simulink model "ADC_Capture_4x4_IQ_DDR4"  (R2019b)
settings: Solver=FixedStepDiscrete  StartTime=0.0  StopTime=inf  RelTol=1e-3
InitFcn:
  | init_ADC_Capture_4x4_IQ_DDR4
values from neighbouring files (symbols this model uses):
  Fs = ConverterSamplingRate/DDC_DUC_factor    (= 512000000)    [init_ADC_Capture_4x4_IQ_DDR4.m]
  N = 14    [init_ADC_Capture_4x4_IQ_DDR4.m]
  sim_CaptureLength = CaptureLength    (= 4096)    [init_ADC_Capture_4x4_IQ_DDR4.m]
  sim_RdFrameSize = 64    [init_ADC_Capture_4x4_IQ_DDR4.m]
  sim_RdNumFrames = ceil(sim_CaptureLength/sim_RdFrameSize)    [init_ADC_Capture_4x4_IQ_DDR4.m]
undefined symbols (not defined in the file or in its folder): config, DDR, Fo
libraries: hdlsllib x35, simulink x20, ddr4_behavioral_mdl x1, AXIDMALib x1, dsphdlsigops x1
(part 2 of 3)

== system ADC_Capture_4x4_IQ_DDR4/HDL_IP/DefaultRegister2 ==
  note: Give it default non-zero value at start-up time
  In1 : Inport
  Compare To Zero : simulink/Logic and Bit Operations/Compare To Zero  relop===  OutDataTypeStr=boolean
  Delay1 : Delay  DelayLength=1
  Switch2 : Switch  Criteria=u2 > Threshold
  range swath cycles : Constant  Value=config.register.range_swath_cycles  OutDataTypeStr=uint32  SampleTime=-1
  Out2 : Outport  VectorParamsAs1DForOutWhenUnconnected=off
  wires:
  In1/1 -> Delay1/1
  range swath cycles/1 -> Switch2/1
  Delay1/1 -> Switch2/3, Compare To Zero/1
  Switch2/1 -> Out2/1
  Compare To Zero/1 -> Switch2/2

== system ADC_Capture_4x4_IQ_DDR4/HDL_IP/DefaultRegister3 ==
  note: Give it default non-zero value at start-up time
  In1 : Inport
  Compare To Zero : simulink/Logic and Bit Operations/Compare To Zero  relop===  OutDataTypeStr=boolean
  Delay1 : Delay  DelayLength=1
  Switch2 : Switch  Criteria=u2 > Threshold
  tx end to rx start cycles : Constant  Value=config.register.tx_end_to_rx_start_delay_cycles  OutDataTypeStr=uint32  SampleTime=-1
  Out2 : Outport  VectorParamsAs1DForOutWhenUnconnected=off
  wires:
  In1/1 -> Delay1/1
  tx end to rx start cycles/1 -> Switch2/1
  Delay1/1 -> Switch2/3, Compare To Zero/1
  Switch2/1 -> Out2/1
  Compare To Zero/1 -> Switch2/2

== system ADC_Capture_4x4_IQ_DDR4/HDL_IP/DefaultRegister4 ==
  note: Give it default non-zero value at start-up time
  In1 : Inport
  Compare To Zero : simulink/Logic and Bit Operations/Compare To Zero  relop===  OutDataTypeStr=boolean
  Constant5 : Constant  Value=config.register.pri_cycles  OutDataTypeStr=uint32  SampleTime=-1
  Delay1 : Delay  DelayLength=1
  Switch2 : Switch  Criteria=u2 > Threshold
  Out2 : Outport  VectorParamsAs1DForOutWhenUnconnected=off
  wires:
  In1/1 -> Delay1/1
  Constant5/1 -> Switch2/1
  Delay1/1 -> Switch2/3, Compare To Zero/1
  Switch2/1 -> Out2/1
  Compare To Zero/1 -> Switch2/2

== system ADC_Capture_4x4_IQ_DDR4/HDL_IP/DefaultRegister5 ==
  note: Give it default non-zero value at start-up time
  In1 : Inport
  Compare To Zero : simulink/Logic and Bit Operations/Compare To Zero  relop===  OutDataTypeStr=boolean
  Constant5 : Constant  Value=config.register.pulse_width_cycles  OutDataTypeStr=uint32  SampleTime=-1
  Delay1 : Delay  DelayLength=1
  Switch2 : Switch  Criteria=u2 > Threshold
  Out2 : Outport  VectorParamsAs1DForOutWhenUnconnected=off
  wires:
  In1/1 -> Delay1/1
  Constant5/1 -> Switch2/1
  Delay1/1 -> Switch2/3, Compare To Zero/1
  Switch2/1 -> Out2/1
  Compare To Zero/1 -> Switch2/2

== system ADC_Capture_4x4_IQ_DDR4/HDL_IP/DefaultRegister6 ==
  note: Give it default non-zero value at start-up time
  In1 : Inport
  Compare To Zero : simulink/Logic and Bit Operations/Compare To Zero  relop===  OutDataTypeStr=boolean
  Constant5 : Constant  Value=config.radar.pulses_per_cpi  OutDataTypeStr=uint32  SampleTime=-1
  Delay1 : Delay  DelayLength=1
  Switch2 : Switch  Criteria=u2 > Threshold
  Out2 : Outport  VectorParamsAs1DForOutWhenUnconnected=off
  wires:
  In1/1 -> Delay1/1
  Constant5/1 -> Switch2/1
  Delay1/1 -> Switch2/3, Compare To Zero/1
  Switch2/1 -> Out2/1
  Compare To Zero/1 -> Switch2/2

== system ADC_Capture_4x4_IQ_DDR4/HDL_IP/DefaultRegister8 ==
  note: Give it default non-zero value at start-up time
  In1 : Inport
  Compare To Zero : simulink/Logic and Bit Operations/Compare To Zero  relop===  OutDataTypeStr=boolean
  Data Type Conversion : DataTypeConversion  OutDataTypeStr=int32
  Delay1 : Delay  DelayLength=1
  Switch2 : Switch  Criteria=u2 > Threshold  OutDataTypeStr=int32
  start inc steps : Constant  Value=config.register.start_inc_steps  OutDataTypeStr=int32
  Out2 : Outport  VectorParamsAs1DForOutWhenUnconnected=off
  wires:
  Compare To Zero/1 -> Switch2/2
  Switch2/1 -> Out2/1
  Delay1/1 -> Compare To Zero/1, Switch2/3
  Data Type Conversion/1 -> Switch2/1
  In1/1 -> Delay1/1
  start inc steps/1 -> Data Type Conversion/1

== system ADC_Capture_4x4_IQ_DDR4/HDL_IP/DefaultRegister9 ==
  note: Give it default non-zero value at start-up time
  In1 : Inport
  Compare To Zero : simulink/Logic and Bit Operations/Compare To Zero  relop===  OutDataTypeStr=boolean
  Data Type Conversion : DataTypeConversion  OutDataTypeStr=int32
  Delay1 : Delay  DelayLength=1
  Switch2 : Switch  Criteria=u2 > Threshold  OutDataTypeStr=int32
  end_inc_steps : Constant  Value=config.register.end_inc_steps  OutDataTypeStr=int32
  Out2 : Outport  VectorParamsAs1DForOutWhenUnconnected=off
  wires:
  Compare To Zero/1 -> Switch2/2
  Switch2/1 -> Out2/1
  Delay1/1 -> Compare To Zero/1, Switch2/3
  Data Type Conversion/1 -> Switch2/1
  In1/1 -> Delay1/1
  end_inc_steps/1 -> Data Type Conversion/1

== system ADC_Capture_4x4_IQ_DDR4/HDL_IP/GateRxData ==
  active : Inport
  in : Inport  Port=2
  Bus Creator : BusCreator  Inputs=3
  Bus Selector4 : BusSelector  OutputSignals=I,Q,Valid
  Delay : Delay  DelayLength=1
  Delay1 : Delay  DelayLength=1
  Delay2 : Delay  DelayLength=1
  Logical Operator : Logic  AllPortsSameDT=off  OutDataTypeStr=boolean
  Signal Conversion13 : SignalConversion  OverrideOpt=off
  Signal Conversion14 : SignalConversion  OverrideOpt=off
  Signal Conversion15 : SignalConversion  OverrideOpt=off
  out : Outport
  wires:
  in/1 -> Delay1/1
  Bus Selector4/3 -> Logical Operator/1  "<Valid>"
  active/1 -> Delay2/1
  Signal Conversion14/1 -> Bus Creator/2  "Q"
  Signal Conversion15/1 -> Bus Creator/3  "Valid"
  Bus Creator/1 -> Delay/1
  Signal Conversion13/1 -> Bus Creator/1  "I"
  Bus Selector4/1 -> Signal Conversion13/1  "<I>"
  Bus Selector4/2 -> Signal Conversion14/1  "<Q>"
  Logical Operator/1 -> Signal Conversion15/1
  Delay/1 -> out/1
  Delay1/1 -> Bus Selector4/1
  Delay2/1 -> Logical Operator/2

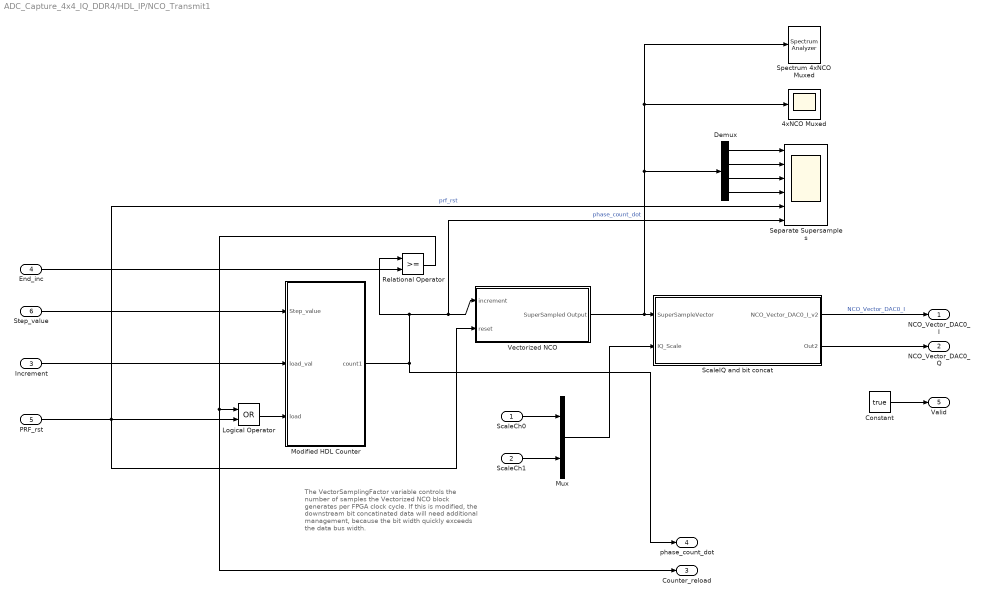
== system ADC_Capture_4x4_IQ_DDR4/HDL_IP/NCO_Transmit1 ==
  note: The VectorSamplingFactor variable controls the
      | number of samples the Vectorized NCO block
      | generates per FPGA clock cycle.
      | If this is modified, the downstream bit concatinated
      | data will need additional management, because
      | the bit width quickly exceeds the data bus width.
  ScaleCh0 : Inport
  ScaleCh1 : Inport  Port=2
  Increment : Inport  Port=3
  End_inc : Inport  Port=4
  PRF_rst : Inport  Port=5
  Step_value : Inport  Port=6
  4xNCO Muxed : Scope
  Constant : Constant  Value=true  SampleTime=-1
  Demux : Demux
  Logical Operator : Logic  Operator=OR  AllPortsSameDT=off  OutDataTypeStr=boolean
  Modified HDL Counter : Subsystem  mask{N=config.synthesis.N_accumulator}
      mask prompts: N "Counter Bit Depth"
      mask init:
      | issigned = 1; % 0 - unsigned, 1 - signed
      | CountInit = 0;
      | CountFracLen = 0;
      | CountWordLen = N;
      | freerun=1;
      | CountFrom = 0;
      | CountDir = 0; % 0-up, 1-down
      | % MaxValue for N bit signed integer
      | MaxValue = 2^(N-1)-1;
  Mux : Mux  Inputs=2
  Relational Operator : RelationalOperator  OutDataTypeStr=boolean  RndMeth=Nearest
  ScaleIQ and bit concat : Subsystem
  Separate Supersamples : Scope  NumInputPorts=6
  Spectrum 4xNCO Muxed : SpectrumAnalyzer
  Vectorized NCO : Subsystem  mask{factor=config.synthesis.samples_per_clock_cycle}
      mask prompts: factor "Vectorization Factor"
      mask init:
      | % Vector of offsets, taken as hidden parameter to block below,
      | % partitioned within for loop
      | % N x 1, so ForEach partition is in dimension 1
      | offsetForEach = [0:factor-1]';
      | 
      | %set_param([gcb '.'], 'vectorOffetTop', '0:factor-1');
  NCO_Vector_DAC0_I : Outport  VectorParamsAs1DForOutWhenUnconnected=off
  NCO_Vector_DAC0_Q : Outport  Port=2  VectorParamsAs1DForOutWhenUnconnected=off
  "Counter_reload " : Outport  Port=3
  phase_count_dot : Outport  Port=4
  "Valid " : Outport  Port=5
  wires:
  Modified HDL Counter/1(count1) -> Relational Operator/1, Separate Supersamples/6, Vectorized NCO/1(increment), phase_count_dot/1  "phase_count_dot"
  Demux/1 -> Separate Supersamples/1
  Demux/2 -> Separate Supersamples/2
  Demux/3 -> Separate Supersamples/3
  Demux/4 -> Separate Supersamples/4
  ScaleCh0/1 -> Mux/1
  ScaleCh1/1 -> Mux/2
  ScaleIQ and bit concat/2(Out2) -> NCO_Vector_DAC0_Q/1
  End_inc/1 -> Relational Operator/2
  Relational Operator/1 -> "Counter_reload "/1, Logical Operator/1
  PRF_rst/1 -> Vectorized NCO/2(reset), Separate Supersamples/5, Logical Operator/2  "prf_rst"
  Step_value/1 -> Modified HDL Counter/1(Step_value)
  Vectorized NCO/1(SuperSampled Output) -> ScaleIQ and bit concat/1(SuperSampleVector), Demux/1, 4xNCO Muxed/1, Spectrum 4xNCO Muxed/1
  Mux/1 -> ScaleIQ and bit concat/2(IQ_Scale)
  ScaleIQ and bit concat/1(NCO_Vector_DAC0_I_v2) -> NCO_Vector_DAC0_I/1  "NCO_Vector_DAC0_I"
  Increment/1 -> Modified HDL Counter/2(load_val)
  Logical Operator/1 -> Modified HDL Counter/3(load)
  Constant/1 -> "Valid "/1

== system ADC_Capture_4x4_IQ_DDR4/HDL_IP/RouteADC ==
  PortSelect : Inport
  Ch0 : Inport  Port=2
  Ch1 : Inport  Port=3
  Ch2 : Inport  Port=4
  Ch3 : Inport  Port=5
  DACDebug : Inport  Port=6
  CounterDebug : Inport  Port=7
  Multiport Switch : MultiPortSwitch  DataPortOrder=Zero-based contiguous  Inputs=8  DataPortForDefault=Additional data port  DiagnosticForDefault=Warning  zeroidx=on
  ChOut : Outport  VectorParamsAs1DForOutWhenUnconnected=off
  wires:
  Ch3/1 -> Multiport Switch/9, Multiport Switch/5
  Ch1/1 -> Multiport Switch/3
  Ch2/1 -> Multiport Switch/8, Multiport Switch/4
  Ch0/1 -> Multiport Switch/10, Multiport Switch/2
  Multiport Switch/1 -> ChOut/1
  PortSelect/1 -> Multiport Switch/1
  DACDebug/1 -> Multiport Switch/6
  CounterDebug/1 -> Multiport Switch/7

== system ADC_Capture_4x4_IQ_DDR4/HDL_IP/Subsystem ==
  note: Verify this delay is still correct...
  I_in : Inport
  Q_in : Inport  Port=2
  ValidIn : Inport  Port=3
  TxActive : Inport  Port=4
  Complex to Real-Imag : ComplexToRealImag
  Constant2 : Constant  Value=complex(0,0)  OutDataTypeStr=Inherit: Inherit via back propagation  SampleTime=-1
  Data Type Duplicate : DataTypeDuplicate
  Delay : Delay  DelayLength=7
  Multiport Switch : MultiPortSwitch  DataPortOrder=Zero-based contiguous  Inputs=2  zeroidx=on
  Real-Imag to Complex : RealImagToComplex
  I_out : Outport
  Q_out : Outport  Port=2
  ValidOut : Outport  Port=3
  wires:
  Real-Imag to Complex/1 -> Multiport Switch/3, Data Type Duplicate/2
  Complex to Real-Imag/1 -> I_out/1
  Complex to Real-Imag/2 -> Q_out/1
  I_in/1 -> Real-Imag to Complex/1
  ValidIn/1 -> ValidOut/1
  TxActive/1 -> Delay/1
  Multiport Switch/1 -> Complex to Real-Imag/1
  Constant2/1 -> Data Type Duplicate/1, Multiport Switch/2
  Q_in/1 -> Real-Imag to Complex/2
  Delay/1 -> Multiport Switch/1

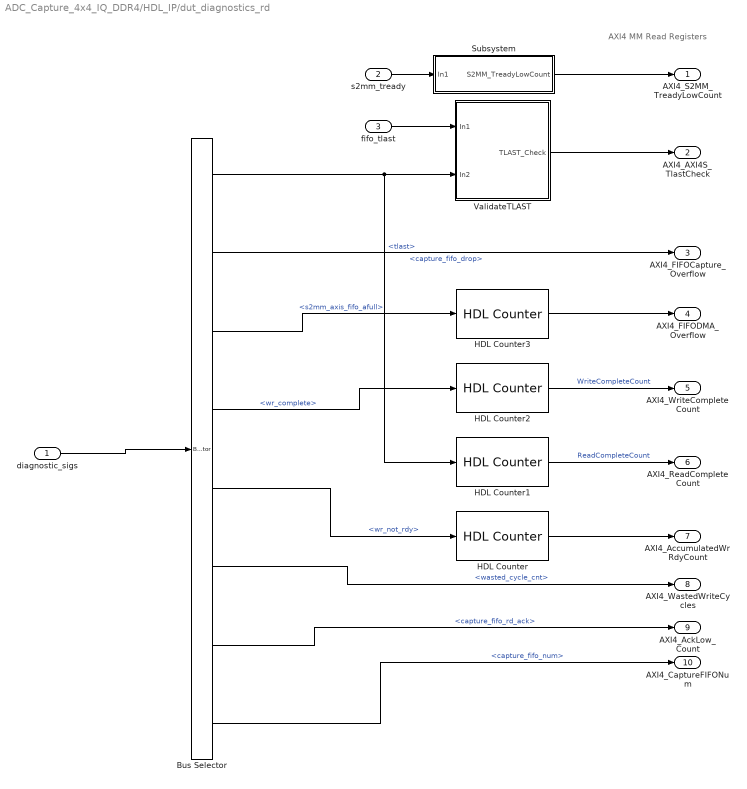
== system ADC_Capture_4x4_IQ_DDR4/HDL_IP/dut_diagnostics_rd ==
  note: AXI4 MM Read Registers
  diagnostic_sigs : Inport
  s2mm_tready : Inport  Port=2
  fifo_tlast : Inport  Port=3
  Bus Selector : BusSelector  OutputSignals=tlast,capture_fifo_drop,s2mm_axis_fifo_afull,wr_complete,wr_not_rdy,wasted_cycle_cnt,capture_fifo_rd_ack,capture_fifo_num
  HDL Counter{,1..3} (4 alike) : hdlsllib/Sources/HDL Counter  CountType=Free running  CountInit=0  CountStep=1  CountMax=25  CountFromType=Initial value  CountFrom=0  CountResetPort=off  CountLoadPort=off  CountEnbPort=on  CountDirPort=off  CountDataType=Unsigned  CountWordLen=32  CountFracLen=0  CountSampTime=1
      settings: SourceProductName=Simulink
  Subsystem : Subsystem
  ValidateTLAST : Subsystem
  AXI4_S2MM_TreadyLowCount : Outport  VectorParamsAs1DForOutWhenUnconnected=off
  AXI4_AXI4S_TlastCheck : Outport  Port=2  VectorParamsAs1DForOutWhenUnconnected=off
  AXI4_FIFOCapture_Overflow : Outport  Port=3  VectorParamsAs1DForOutWhenUnconnected=off
  AXI4_FIFODMA_Overflow : Outport  Port=4  VectorParamsAs1DForOutWhenUnconnected=off
  AXI4_WriteCompleteCount : Outport  Port=5  VectorParamsAs1DForOutWhenUnconnected=off
  AXI4_ReadCompleteCount : Outport  Port=6  VectorParamsAs1DForOutWhenUnconnected=off
  AXI4_AccumulatedWrRdyCount : Outport  Port=7  VectorParamsAs1DForOutWhenUnconnected=off
  AXI4_WastedWriteCycles : Outport  Port=8  VectorParamsAs1DForOutWhenUnconnected=off
  AXI4_AckLow_Count : Outport  Port=9  VectorParamsAs1DForOutWhenUnconnected=off
  AXI4_CaptureFIFONum : Outport  Port=10  VectorParamsAs1DForOutWhenUnconnected=off
  wires:
  diagnostic_sigs/1 -> Bus Selector/1
  Bus Selector/8 -> AXI4_CaptureFIFONum/1  "<capture_fifo_num>"
  HDL Counter1/1 -> AXI4_ReadCompleteCount/1  "ReadCompleteCount"
  HDL Counter/1 -> AXI4_AccumulatedWrRdyCount/1
  ValidateTLAST/1(TLAST_Check) -> AXI4_AXI4S_TlastCheck/1
  HDL Counter3/1 -> AXI4_FIFODMA_Overflow/1
  Bus Selector/6 -> AXI4_WastedWriteCycles/1  "<wasted_cycle_cnt>"
  HDL Counter2/1 -> AXI4_WriteCompleteCount/1  "WriteCompleteCount"
  Subsystem/1(S2MM_TreadyLowCount) -> AXI4_S2MM_TreadyLowCount/1
  s2mm_tready/1 -> Subsystem/1(In1)
  fifo_tlast/1 -> ValidateTLAST/1(In1)
  Bus Selector/1 -> HDL Counter1/1, ValidateTLAST/2(In2)  "<tlast>"
  Bus Selector/3 -> HDL Counter3/1  "<s2mm_axis_fifo_afull>"
  Bus Selector/4 -> HDL Counter2/1  "<wr_complete>"
  Bus Selector/5 -> HDL Counter/1  "<wr_not_rdy>"
  Bus Selector/7 -> AXI4_AckLow_Count/1  "<capture_fifo_rd_ack>"
  Bus Selector/2 -> AXI4_FIFOCapture_Overflow/1  "<capture_fifo_drop>"

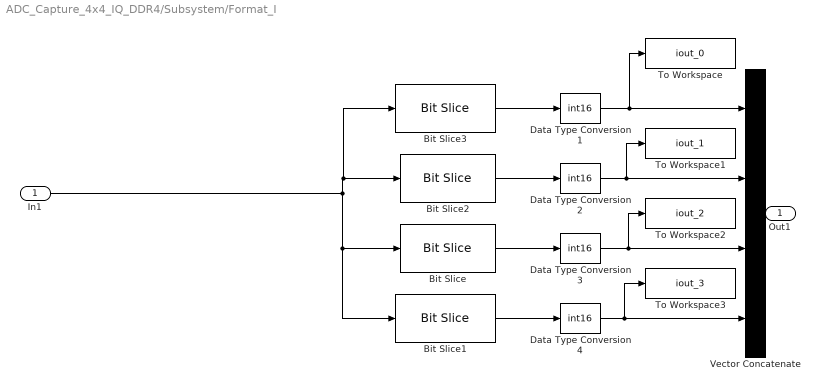
== system ADC_Capture_4x4_IQ_DDR4/Subsystem/Format_I ==
  In1 : Inport
  Bit Slice : hdlsllib/Logic and Bit Operations/Bit Slice  lidx=47  ridx=32
  Bit Slice1 : hdlsllib/Logic and Bit Operations/Bit Slice  lidx=63  ridx=48
  Bit Slice2 : hdlsllib/Logic and Bit Operations/Bit Slice  lidx=31  ridx=16
  Bit Slice3 : hdlsllib/Logic and Bit Operations/Bit Slice  lidx=15  ridx=0
  Data Type Conversion{1..4} (4 alike) : DataTypeConversion  OutDataTypeStr=int16  ConvertRealWorld=Stored Integer (SI)
  To Workspace : ToWorkspace  VariableName=iout_0  SaveFormat=Timeseries  SampleTime=-1
  To Workspace1 : ToWorkspace  VariableName=iout_1  SaveFormat=Timeseries  SampleTime=-1
  To Workspace2 : ToWorkspace  VariableName=iout_2  SaveFormat=Timeseries  SampleTime=-1
  To Workspace3 : ToWorkspace  VariableName=iout_3  SaveFormat=Timeseries  SampleTime=-1
  Vector Concatenate : Concatenate  NumInputs=4  Mode=Multidimensional array
  Out1 : Outport  VectorParamsAs1DForOutWhenUnconnected=off
  wires:
  In1/1 -> Bit Slice1/1, Bit Slice/1, Bit Slice3/1, Bit Slice2/1
  Bit Slice3/1 -> Data Type Conversion1/1
  Data Type Conversion4/1 -> To Workspace3/1, Vector Concatenate/4
  Data Type Conversion3/1 -> To Workspace2/1, Vector Concatenate/3
  Data Type Conversion1/1 -> To Workspace/1, Vector Concatenate/1
  Bit Slice1/1 -> Data Type Conversion4/1
  Bit Slice/1 -> Data Type Conversion3/1
  Vector Concatenate/1 -> Out1/1
  Bit Slice2/1 -> Data Type Conversion2/1
  Data Type Conversion2/1 -> To Workspace1/1, Vector Concatenate/2

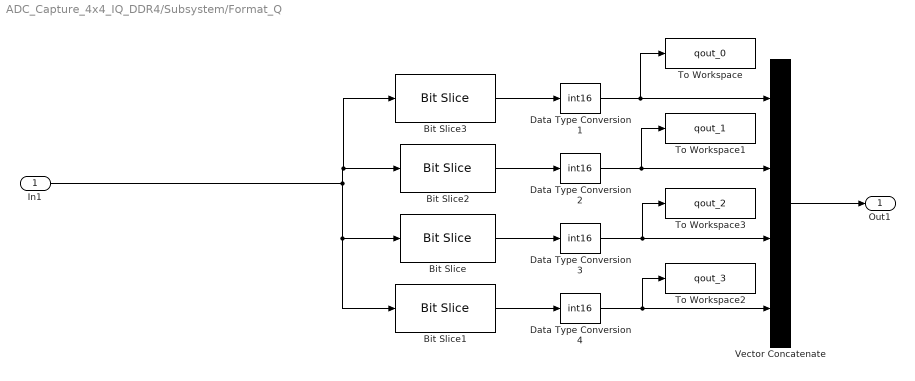
== system ADC_Capture_4x4_IQ_DDR4/Subsystem/Format_Q ==
  In1 : Inport
  Bit Slice : hdlsllib/Logic and Bit Operations/Bit Slice  lidx=47  ridx=32
  Bit Slice1 : hdlsllib/Logic and Bit Operations/Bit Slice  lidx=63  ridx=48
  Bit Slice2 : hdlsllib/Logic and Bit Operations/Bit Slice  lidx=31  ridx=16
  Bit Slice3 : hdlsllib/Logic and Bit Operations/Bit Slice  lidx=15  ridx=0
  Data Type Conversion{1..4} (4 alike) : DataTypeConversion  OutDataTypeStr=int16  ConvertRealWorld=Stored Integer (SI)
  To Workspace : ToWorkspace  VariableName=qout_0  SaveFormat=Timeseries  SampleTime=-1
  To Workspace1 : ToWorkspace  VariableName=qout_1  SaveFormat=Timeseries  SampleTime=-1
  To Workspace2 : ToWorkspace  VariableName=qout_3  SaveFormat=Timeseries  SampleTime=-1
  To Workspace3 : ToWorkspace  VariableName=qout_2  SaveFormat=Timeseries  SampleTime=-1
  Vector Concatenate : Concatenate  NumInputs=4  Mode=Multidimensional array
  Out1 : Outport  VectorParamsAs1DForOutWhenUnconnected=off
  wires:
  In1/1 -> Bit Slice1/1, Bit Slice/1, Bit Slice3/1, Bit Slice2/1
  Bit Slice3/1 -> Data Type Conversion1/1
  Data Type Conversion4/1 -> To Workspace2/1, Vector Concatenate/4
  Data Type Conversion3/1 -> To Workspace3/1, Vector Concatenate/3
  Data Type Conversion1/1 -> To Workspace/1, Vector Concatenate/1
  Bit Slice1/1 -> Data Type Conversion4/1
  Bit Slice/1 -> Data Type Conversion3/1
  Data Type Conversion2/1 -> To Workspace1/1, Vector Concatenate/2
  Vector Concatenate/1 -> Out1/1
  Bit Slice2/1 -> Data Type Conversion2/1

== system ADC_Capture_4x4_IQ_DDR4/DDR4 Model/DDR3/ddr_ready ==
  Enable : EnablePort
  Data Type Conversion : DataTypeConversion  OutDataTypeStr=boolean
  Pulse Generator : DiscretePulseGenerator  Period=1000  PulseWidth=1000 * READY_DUTY_CYL  SampleTime=-1
  rdy_out : Outport  VectorParamsAs1DForOutWhenUnconnected=off
  wires:
  Pulse Generator/1 -> Data Type Conversion/1
  Data Type Conversion/1 -> rdy_out/1

== system ADC_Capture_4x4_IQ_DDR4/DDR4 Model/DDR3/rdLogic ==
  axim_rd_addr : Inport
  axim_rd_len : Inport  Port=2
  axim_rd_avalid : Inport  Port=3
  axi_rd_dready : Inport  Port=4
  Bit Slice1 : hdlsllib/Logic and Bit Operations/Bit Slice  lidx=15  ridx=0
  Constant : Constant  OutDataTypeStr=boolean  SampleTime=-1
  Delay2 : Delay
  rd_control : MATLAB Function  TreatAsAtomicUnit=on
  ram_rd_addr : Outport  VectorParamsAs1DForOutWhenUnconnected=off
  axim_rd_aready : Outport  Port=2  VectorParamsAs1DForOutWhenUnconnected=off
  axim_rd_dvalid : Outport  Port=3  VectorParamsAs1DForOutWhenUnconnected=off
  wires:
  axim_rd_addr/1 -> rd_control/1(axi_rd_add)
  rd_control/1(ram_rd_addr) -> Bit Slice1/1
  axim_rd_avalid/1 -> rd_control/3(axi_rd_val)
  Bit Slice1/1 -> ram_rd_addr/1
  axi_rd_dready/1 -> rd_control/4(axi_rd_ready)
  Delay2/1 -> axim_rd_dvalid/1
  Constant/1 -> axim_rd_aready/1
  axim_rd_len/1 -> rd_control/2(axi_rd_len)
  rd_control/2(ram_rd_val) -> Delay2/1

== system ADC_Capture_4x4_IQ_DDR4/DDR4 Model/DDR3/wrLogic ==
  ddr_rdy : Inport
  axi_addr : Inport  Port=2
  axi_wr_len : Inport  Port=3
  axi_wr_enb : Inport  Port=4
  Add : Sum  AccumDataTypeStr=uint32
  Bit Shift : hdlsllib/Logic and Bit Operations/Bit Shift  mode=Shift Right Arithmetic  N=log2(WR_RD_DATAWIDTH/8)
      settings: SourceProductName=HDL Coder  SourceProductBaseCode=HD
  Logical Operator : Logic  Operator=OR  IconShape=distinctive  AllPortsSameDT=off  OutDataTypeStr=boolean
  Wr_control : Subsystem
  ddr_ack_d1 : Delay  DelayLength=1
  ddr_reday_d1 : Delay  DelayLength=1
  ddr_reday_d6 : Delay  DelayLength=4
  ram_wr_addr : Outport  VectorParamsAs1DForOutWhenUnconnected=off
  ram_wr_enb : Outport  Port=2  VectorParamsAs1DForOutWhenUnconnected=off
  axi_wr_ack : Outport  Port=3  VectorParamsAs1DForOutWhenUnconnected=off
  wires:
  Wr_control/1(valAddEnb) -> ram_wr_enb/1
  axi_wr_len/1 -> Wr_control/3(wr_len)
  ddr_rdy/1 -> ddr_reday_d6/1
  axi_wr_enb/1 -> Wr_control/2(wr_enb)
  Wr_control/2(axim_ack) -> ddr_ack_d1/1
  Add/1 -> ram_wr_addr/1
  Wr_control/3(ram_addr) -> Add/2
  ddr_reday_d6/1 -> ddr_reday_d1/1, Logical Operator/2
  ddr_ack_d1/1 -> axi_wr_ack/1
  axi_addr/1 -> Bit Shift/1
  ddr_reday_d1/1 -> Logical Operator/1
  Logical Operator/1 -> Wr_control/1(ddr_wr_rdy)
  Bit Shift/1 -> Add/1

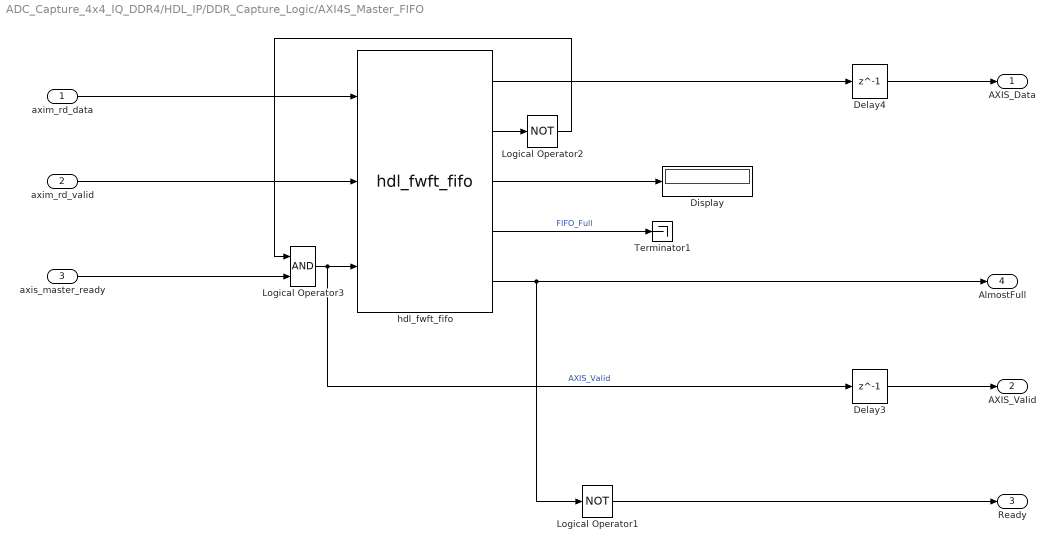
== system ADC_Capture_4x4_IQ_DDR4/HDL_IP/DDR_Capture_Logic/AXI4S_Master_FIFO  ==
  axim_rd_data : Inport
  axim_rd_valid : Inport  Port=2
  axis_master_ready : Inport  Port=3
  Delay3 : Delay  DelayLength=1
  Delay4 : Delay  DelayLength=1
  Display : Display
  Logical Operator1 : Logic  Operator=NOT  IconShape=distinctive  AllPortsSameDT=off  OutDataTypeStr=boolean
  Logical Operator2 : Logic  Operator=NOT  IconShape=distinctive  AllPortsSameDT=off  OutDataTypeStr=boolean
  Logical Operator3 : Logic  IconShape=distinctive  AllPortsSameDT=off  OutDataTypeStr=boolean
  Terminator1 : Terminator
  hdl_fwft_fifo : AXIDMALib/Hardware/hdl_fwft_fifo  FIFO_DEPTH=5*1024  AFULL_THRESH=ceil(5*1024*0.1)
  AXIS_Data : Outport  VectorParamsAs1DForOutWhenUnconnected=off
  AXIS_Valid : Outport  Port=2  VectorParamsAs1DForOutWhenUnconnected=off
  Ready : Outport  Port=3  VectorParamsAs1DForOutWhenUnconnected=off
  AlmostFull : Outport  Port=4  VectorParamsAs1DForOutWhenUnconnected=off
  wires:
  Logical Operator3/1 -> Delay3/1, hdl_fwft_fifo/3  "AXIS_Valid"
  axim_rd_valid/1 -> hdl_fwft_fifo/2
  hdl_fwft_fifo/2 -> Logical Operator2/1
  Logical Operator2/1 -> Logical Operator3/1
  hdl_fwft_fifo/3 -> Display/1
  hdl_fwft_fifo/4 -> Terminator1/1  "FIFO_Full"
  axim_rd_data/1 -> hdl_fwft_fifo/1
  axis_master_ready/1 -> Logical Operator3/2
  hdl_fwft_fifo/1 -> Delay4/1
  Delay4/1 -> AXIS_Data/1
  Logical Operator1/1 -> Ready/1
  hdl_fwft_fifo/5 -> AlmostFull/1, Logical Operator1/1
  Delay3/1 -> AXIS_Valid/1

== system ADC_Capture_4x4_IQ_DDR4/HDL_IP/DDR_Capture_Logic/DataBusBreakout ==
  busIn : Inport
  Bit Concat1 : hdlsllib/Logic and Bit Operations/Bit Concat  numInputs=2
      settings: SourceProductName=Simulink
  Bus Selector3 : BusSelector  OutputSignals=Q,I,Valid
  dataOut : Outport
  validOut : Outport  Port=2
  wires:
  Bus Selector3/2 -> Bit Concat1/2  "<I>"
  Bus Selector3/1 -> Bit Concat1/1  "<Q>"
  busIn/1 -> Bus Selector3/1
  Bus Selector3/3 -> validOut/1  "<Valid>"
  Bit Concat1/1 -> dataOut/1

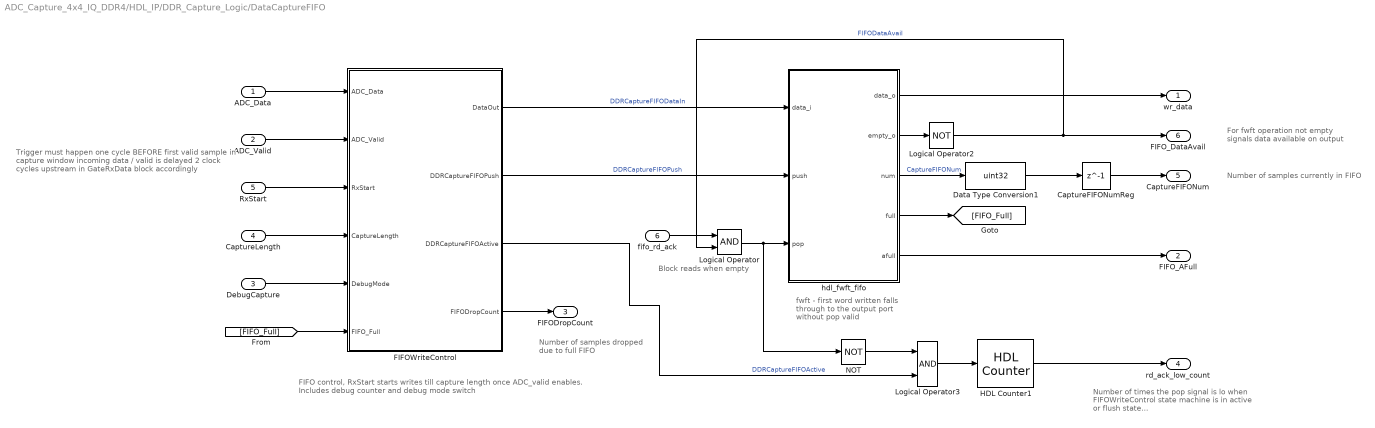
== system ADC_Capture_4x4_IQ_DDR4/HDL_IP/DDR_Capture_Logic/DataCaptureFIFO ==
  note: Number of samples dropped
      | due to full FIFO
  note: Number of samples currently in FIFO
  note: Number of times the pop signal is
      | lo when FIFOWriteControl state machine
      | is in active or flush state...
  note: For fwft operation not empty
      | signals data available on output
  note: Block reads when empty
  note: fwft - first word written falls
      | through to the output port
      | without pop valid
  note: FIFO control, RxStart starts writes till capture length once ADC_valid enables.
      |  Includes debug counter and debug mode switch
  note: Trigger must happen one cycle BEFORE
      | first valid sample in capture window incoming
      | data / valid is delayed 2 clock cycles upstream
      | in GateRxData block accordingly
  ADC_Data : Inport
  ADC_Valid : Inport  Port=2
  DebugCapture : Inport  Port=3
  CaptureLength : Inport  Port=4
  RxStart : Inport  Port=5
  fifo_rd_ack : Inport  Port=6
  CaptureFIFONumReg : Delay  DelayLength=1
  Data Type Conversion1 : DataTypeConversion  OutDataTypeStr=uint32
  FIFOWriteControl : Subsystem
      settings: PortSchema="{\"entries\":[{\"content\":{\"sides\":[{\"content\":{\"connectorIds\":[\"In1\",\"In2\",\"In3\",\"In4\",\"In5\",\"In6\"]},\"type\":\"ConnectorPlacement.EquallySpacedRectSide\",\"uuid\":\"e521c4e1-d63e-4776-a5fe-9169b813b24e\"},{\"content\":{\"connectorIds\":[\"Out1\",\"Out2\",\"Out3\",\"Out4\"],\"side\":\"RIGHT\"},\"type\":\"ConnectorPlacement.EquallySpacedRectSide\",\"uuid\":\"3008809a-f1e7-4909-9ea3-d872427f328e\"},{\"content\":{\"connectorIds\":[],\"side\":\"TOP\"},\"type\":\"ConnectorPlacement.EquallySpacedRectSide\",\"uuid\":\"bb3d8776-800b-4946-a7b2-f09ccb0b78e9\"}]},\"type\":\"ConnectorPlacement.EquallySpacedConnector\",\"uuid\":\"eeb97d5f-4442-4cf8-a47a-4f33546d9dbc\"}],\"packageUris\":[\"http://schema.mathworks.com/mf0/Connector/19700101\"],\"version\":\"1.0\"}"
  HDL Counter1 : hdlsllib/Sources/HDL Counter  CountType=Free running  CountInit=0  CountStep=1  CountMax=25  CountFromType=Initial value  CountFrom=0  CountResetPort=off  CountLoadPort=off  CountEnbPort=on  CountDirPort=off  CountDataType=Unsigned  CountWordLen=32  CountFracLen=0  CountSampTime=1
      settings: SourceProductBaseCode=HD
  Logical Operator : Logic  AllPortsSameDT=off  OutDataTypeStr=boolean
  Logical Operator2 : Logic  Operator=NOT  IconShape=distinctive  AllPortsSameDT=off  OutDataTypeStr=boolean
  Logical Operator3 : Logic  AllPortsSameDT=off  OutDataTypeStr=boolean
  NOT : Logic  Operator=NOT  IconShape=distinctive  AllPortsSameDT=off  OutDataTypeStr=boolean
  hdl_fwft_fifo : Subsystem  mask{FIFO_DEPTH=10*1024, AFULL_THRESH=1024}
      mask prompts: FIFO_DEPTH "FIFO Depth"; AFULL_THRESH "Almost Full Threshold"
      mask init:
      | FIFO_CNT_BITS=ceil(log2(FIFO_DEPTH+1+3));
  wr_data : Outport  VectorParamsAs1DForOutWhenUnconnected=off
  FIFO_AFull : Outport  Port=2  VectorParamsAs1DForOutWhenUnconnected=off
  FIFODropCount : Outport  Port=3  VectorParamsAs1DForOutWhenUnconnected=off
  rd_ack_low_count : Outport  Port=4  VectorParamsAs1DForOutWhenUnconnected=off
  CaptureFIFONum : Outport  Port=5  VectorParamsAs1DForOutWhenUnconnected=off
  FIFO_DataAvail : Outport  Port=6  VectorParamsAs1DForOutWhenUnconnected=off
  wires:
  hdl_fwft_fifo/3(num) -> Data Type Conversion1/1  "CaptureFIFONum"
  hdl_fwft_fifo/2(empty_o) -> Logical Operator2/1
  Logical Operator2/1 -> Logical Operator/2, FIFO_DataAvail/1  "FIFODataAvail"
  FIFOWriteControl/2(DDRCaptureFIFOPush) -> hdl_fwft_fifo/2(push)  "DDRCaptureFIFOPush"
  hdl_fwft_fifo/5(afull) -> FIFO_AFull/1
  hdl_fwft_fifo/1(data_o) -> wr_data/1
  FIFOWriteControl/1(DataOut) -> hdl_fwft_fifo/1(data_i)  "DDRCaptureFIFODataIn"
  Logical Operator/1 -> hdl_fwft_fifo/3(pop), NOT/1
  fifo_rd_ack/1 -> Logical Operator/1
  NOT/1 -> Logical Operator3/1
  Logical Operator3/1 -> HDL Counter1/1
  HDL Counter1/1 -> rd_ack_low_count/1
  Data Type Conversion1/1 -> CaptureFIFONumReg/1
  CaptureFIFONumReg/1 -> CaptureFIFONum/1
  RxStart/1 -> FIFOWriteControl/3(RxStart)
  ADC_Valid/1 -> FIFOWriteControl/2(ADC_Valid)
  ADC_Data/1 -> FIFOWriteControl/1(ADC_Data)
  FIFOWriteControl/3(DDRCaptureFIFOActive) -> Logical Operator3/2  "DDRCaptureFIFOActive"
  hdl_fwft_fifo/4(full) -> [FIFO_Full]
  CaptureLength/1 -> FIFOWriteControl/4(CaptureLength)
  DebugCapture/1 -> FIFOWriteControl/5(DebugMode)
  [FIFO_Full] -> FIFOWriteControl/6(FIFO_Full)
  FIFOWriteControl/4(FIFODropCount) -> FIFODropCount/1

== system ADC_Capture_4x4_IQ_DDR4/HDL_IP/DDR_Capture_Logic/TLAST_Align ==
  axim_rd_data : Inport
  axim_rd_valid : Inport  Port=2
  axis_master_ready : Inport  Port=3
  Delay3 : Delay  DelayLength=1
  Delay4 : Delay  DelayLength=1
  Display : Display
  HDL FIFO : hdlsllib/HDL RAMs/HDL FIFO  fifo_size=5*1024  mode=FWFT  ratio=1  push_msg=Warning  pop_msg=Warning  show_empty=on  show_full=on  show_num=on  LabelModeActiveChoice_Mode=FWFT
      settings: SourceProductName=Simulink  SourceProductBaseCode=SL
  Logical Operator2 : Logic  Operator=NOT  IconShape=distinctive  AllPortsSameDT=off  OutDataTypeStr=boolean
  Logical Operator3 : Logic  IconShape=distinctive  AllPortsSameDT=off  OutDataTypeStr=boolean
  Terminator1 : Terminator
  AXIS_Data : Outport  VectorParamsAs1DForOutWhenUnconnected=off
  AXIS_Valid : Outport  Port=2  VectorParamsAs1DForOutWhenUnconnected=off
  wires:
  Logical Operator3/1 -> Delay3/1, HDL FIFO/3  "AXIS_Valid"
  HDL FIFO/2 -> Logical Operator2/1
  Logical Operator2/1 -> Logical Operator3/1
  HDL FIFO/3 -> Display/1
  HDL FIFO/4 -> Terminator1/1  "FIFO_Full"
  axim_rd_data/1 -> HDL FIFO/1
  axis_master_ready/1 -> Logical Operator3/2
  HDL FIFO/1 -> Delay4/1
  Delay4/1 -> AXIS_Data/1
  Delay3/1 -> AXIS_Valid/1
  axim_rd_valid/1 -> HDL FIFO/2

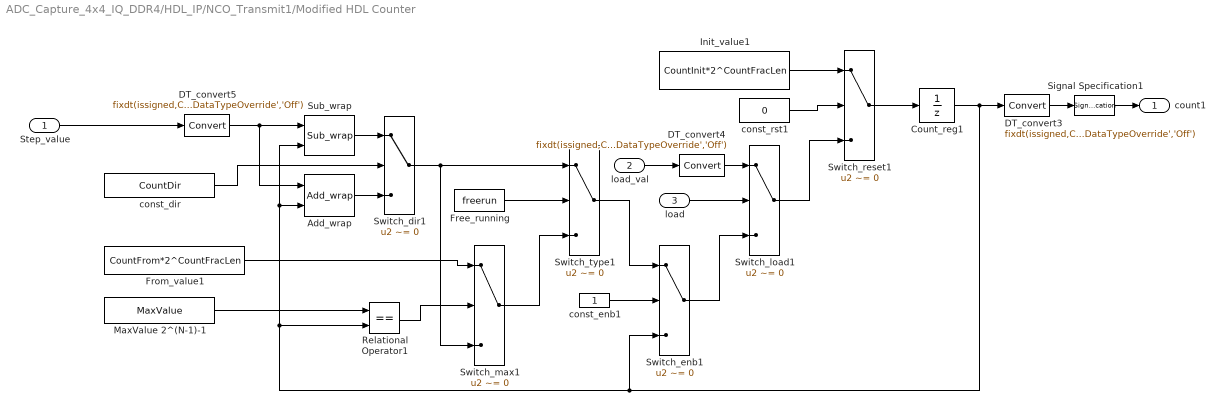
== system ADC_Capture_4x4_IQ_DDR4/HDL_IP/NCO_Transmit1/Modified HDL Counter ==
  Step_value : Inport  PortDimensions=1
  load_val : Inport  Port=2  PortDimensions=1
  load : Inport  Port=3  OutDataTypeStr=boolean  PortDimensions=1
  Add_wrap : hdlsllib/Sources/HDL Counter/Add_wrap  SystemSampleTime=-1  Latency=0  AutoFrameSizeCalculation=off
      settings: SourceProductName=Simulink  SourceProductBaseCode=SL
  Count_reg1 : UnitDelay  InitialCondition=CountInit*2^CountFracLen  SampleTime=-1  HasFrameUpgradeWarning=on
  DT_convert3 : DataTypeConversion  OutDataTypeStr=fixdt(issigned,CountWordLen,CountFracLen,'DataTypeOverride','Off')  ConvertRealWorld=Stored Integer (SI)
  DT_convert4 : DataTypeConversion  OutDataTypeStr=fixdt(issigned,CountWordLen,0,'DataTypeOverride','Off')  ConvertRealWorld=Stored Integer (SI)
  DT_convert5 : DataTypeConversion  OutDataTypeStr=fixdt(issigned,CountWordLen,CountFracLen,'DataTypeOverride','Off')  ConvertRealWorld=Stored Integer (SI)
  Free_running : Constant  Value=freerun  OutDataTypeStr=boolean
  From_value1 : Constant  Value=CountFrom*2^CountFracLen  OutDataTypeStr=fixdt(issigned,CountWordLen, 0,'DataTypeOverride','Off')
  Init_value1 : Constant  Value=CountInit*2^CountFracLen  OutDataTypeStr=fixdt(issigned,CountWordLen, 0,'DataTypeOverride','Off')
  MaxValue 2^(N-1)-1 : Constant  Value=MaxValue  OutDataTypeStr=Inherit: Inherit via back propagation
  Relational Operator1 : RelationalOperator  Operator===  OutDataTypeStr=boolean  RndMeth=Nearest
  Signal Specification1 : SignalSpecification  Dimensions=1
  Sub_wrap : hdlsllib/Sources/HDL Counter/Sub_wrap  SystemSampleTime=-1  Latency=0  AutoFrameSizeCalculation=off
      settings: SourceProductName=Simulink  SourceProductBaseCode=SL
  Switch_dir1 : Switch  Criteria=u2 ~= 0
  Switch_enb1 : Switch  Criteria=u2 ~= 0
  Switch_load1 : Switch  Criteria=u2 ~= 0
  Switch_max1 : Switch  Criteria=u2 ~= 0
  Switch_reset1 : Switch  Criteria=u2 ~= 0  OutDataTypeStr=fixdt(issigned,CountWordLen, 0,'DataTypeOverride','Off')
  Switch_type1 : Switch  Criteria=u2 ~= 0
  const_dir : Constant  Value=CountDir  OutDataTypeStr=boolean
  const_enb1 : Constant  OutDataTypeStr=boolean
  const_rst1 : Constant  Value=0  OutDataTypeStr=boolean
  count1 : Outport  VectorParamsAs1DForOutWhenUnconnected=off
  wires:
  MaxValue 2^(N-1)-1/1 -> Relational Operator1/1
  Step_value/1 -> DT_convert5/1
  DT_convert5/1 -> Sub_wrap/1, Add_wrap/1
  const_rst1/1 -> Switch_reset1/2
  From_value1/1 -> Switch_max1/1
  Switch_max1/1 -> Switch_type1/3
  Relational Operator1/1 -> Switch_max1/2
  load_val/1 -> DT_convert4/1
  Free_running/1 -> Switch_type1/2
  Init_value1/1 -> Switch_reset1/1
  Switch_reset1/1 -> Count_reg1/1
  Count_reg1/1 -> DT_convert3/1, Add_wrap/2, Sub_wrap/2, Relational Operator1/2, Switch_enb1/3
  Switch_type1/1 -> Switch_enb1/1
  DT_convert3/1 -> Signal Specification1/1
  Switch_enb1/1 -> Switch_load1/3
  Switch_load1/1 -> Switch_reset1/3
  const_enb1/1 -> Switch_enb1/2
  Add_wrap/1 -> Switch_dir1/3
  load/1 -> Switch_load1/2
  DT_convert4/1 -> Switch_load1/1
  Signal Specification1/1 -> count1/1
  Sub_wrap/1 -> Switch_dir1/1
  Switch_dir1/1 -> Switch_max1/3, Switch_type1/1
  const_dir/1 -> Switch_dir1/2

== system ADC_Capture_4x4_IQ_DDR4/HDL_IP/NCO_Transmit1/ScaleIQ and bit concat ==
  note: Bit concatenate super sampled vector for ADC.
      | Multiple Samples per FPGA clock.
  note: Apply I_Scale and Q_Scale
      | to vector of complex signals
  SuperSampleVector : Inport
  IQ_Scale : Inport  Port=2
  Bit Concat : hdlsllib/Logic and Bit Operations/Bit Concat  numInputs=1
      settings: SourceProductName=Simulink
  Bit Concat1 : hdlsllib/Logic and Bit Operations/Bit Concat  numInputs=1
      settings: SourceProductName=Simulink
  Demux1 : Demux  Outputs=2
  For Each IQ Scale : Subsystem  TreatAsAtomicUnit=on
  HDL Flip1 : MATLAB Function  TreatAsAtomicUnit=on
  HDL Flip2 : MATLAB Function  TreatAsAtomicUnit=on
  NCO_Vector_DAC0_I_v2 : Outport
  Out2 : Outport  Port=2
  wires:
  HDL Flip2/1(y) -> Bit Concat1/1
  For Each IQ Scale/1(ScaledSample_I) -> HDL Flip1/1(u)
  For Each IQ Scale/2(ScaledSample_Q) -> HDL Flip2/1(u)
  Demux1/2 -> For Each IQ Scale/3(Scale_Q)
  HDL Flip1/1(y) -> Bit Concat/1
  Bit Concat1/1 -> Out2/1
  Demux1/1 -> For Each IQ Scale/2(Scale_I)
  SuperSampleVector/1 -> For Each IQ Scale/1(SampleVector)
  IQ_Scale/1 -> Demux1/1
  Bit Concat/1 -> NCO_Vector_DAC0_I_v2/1  "NCO_Vector_DAC0_I_v2"

== system ADC_Capture_4x4_IQ_DDR4/HDL_IP/NCO_Transmit1/Vectorized NCO ==
  note: Vectorized NCO
      | Inner Mask
  increment : Inport
  reset : Inport  Port=2
  For Each NCO Vectorized : Subsystem  TreatAsAtomicUnit=on
  Gain : Gain  Gain=factor  OutDataTypeStr=Inherit: Inherit via back propagation  ParamDataTypeStr=Inherit: Same as input
  Gain3 : Gain  Gain=offsetForEach  OutDataTypeStr=Inherit: Inherit via back propagation
  SuperSampled Output : Outport
  wires:
  For Each NCO Vectorized/1(ComplexChirp Vectorized Samples) -> SuperSampled Output/1
  increment/1 -> Gain/1, Gain3/1
  Gain/1 -> For Each NCO Vectorized/1(inc)
  Gain3/1 -> For Each NCO Vectorized/2(offset)
  reset/1 -> For Each NCO Vectorized/3(reset)

== system ADC_Capture_4x4_IQ_DDR4/HDL_IP/dut_diagnostics_rd/Subsystem ==
  In1 : Inport
  Add : Sum  OutDataTypeStr=uint32
  Compare To Zero : simulink/Logic and Bit Operations/Compare To Zero  relop===  OutDataTypeStr=boolean
  Data Type Conversion3 : DataTypeConversion  OutDataTypeStr=uint32
  Delay18 : Delay  DelayLength=1
  S2MM_TreadyLowCount : Outport  VectorParamsAs1DForOutWhenUnconnected=off
  wires:
  Compare To Zero/1 -> Data Type Conversion3/1
  Delay18/1 -> S2MM_TreadyLowCount/1, Add/2
  In1/1 -> Compare To Zero/1
  Add/1 -> Delay18/1
  Data Type Conversion3/1 -> Add/1

== system ADC_Capture_4x4_IQ_DDR4/HDL_IP/dut_diagnostics_rd/ValidateTLAST ==
  note: Check to see if TLAST pulse got lost in the FIFO
      | due to overflows. If there is a constant difference then it means TLAST
      | was dropped due to back-pressure and the FIFO filling up to capacity. The AXIS
      | frame is now corrupted
  In1 : Inport
  In2 : Inport  Port=2
  Add : Sum  AccumDataTypeStr=uint32
  Add1 : Sum  AccumDataTypeStr=uint32
  Add2 : Sum  Inputs=+-  AccumDataTypeStr=int32
  Data Type Conversion3 : DataTypeConversion  OutDataTypeStr=uint32
  Data Type Conversion4 : DataTypeConversion  OutDataTypeStr=uint32
  Delay{1..5} (5 alike) : Delay  DelayLength=1
  Detect Increase : simulink/Logic and Bit Operations/Detect Increase  vinit=0.0  OutDataTypeStr=boolean
  Detect Increase1 : simulink/Logic and Bit Operations/Detect Increase  vinit=0.0  OutDataTypeStr=boolean
  TLAST_Check : Outport  VectorParamsAs1DForOutWhenUnconnected=off
  wires:
  Data Type Conversion3/1 -> Add/1
  Data Type Conversion4/1 -> Add1/1
  Delay1/1 -> Add/2, Add2/1
  Add/1 -> Delay1/1
  In2/1 -> Delay4/1
  Delay2/1 -> Add1/2, Add2/2
  In1/1 -> Delay3/1
  Add1/1 -> Delay2/1
  Add2/1 -> Delay5/1
  Detect Increase/1 -> Data Type Conversion3/1
  Detect Increase1/1 -> Data Type Conversion4/1
  Delay3/1 -> Detect Increase/1
  Delay4/1 -> Detect Increase1/1
  Delay5/1 -> TLAST_Check/1

== system ADC_Capture_4x4_IQ_DDR4/DDR4 Model/DDR3/wrLogic/Wr_control ==
  ddr_wr_rdy : Inport
  wr_enb : Inport  Port=2
  wr_len : Inport  Port=3
  AckGen : Subsystem
  MATLAB Function : MATLAB Function  TreatAsAtomicUnit=on
  Unit Delay : UnitDelay  SampleTime=-1  HasFrameUpgradeWarning=on
  valAddEnb : Outport  VectorParamsAs1DForOutWhenUnconnected=off
  axim_ack : Outport  Port=2  VectorParamsAs1DForOutWhenUnconnected=off
  ram_addr : Outport  Port=3  VectorParamsAs1DForOutWhenUnconnected=off
  wires:
  wr_enb/1 -> AckGen/2(wrEnb), MATLAB Function/1(axi_wr_en)
  AckGen/2(ValAddEnb) -> valAddEnb/1
  wr_len/1 -> MATLAB Function/2(axi_wr_length)
  AckGen/1(ack) -> Unit Delay/1
  MATLAB Function/1(wr_leng) -> AckGen/1(axiWrLen)
  Unit Delay/1 -> axim_ack/1, MATLAB Function/3(wr_ack)
  AckGen/3(ram_addr) -> ram_addr/1
  ddr_wr_rdy/1 -> AckGen/3(ddr_wr_rdy)

== system ADC_Capture_4x4_IQ_DDR4/HDL_IP/DDR_Capture_Logic/DataCaptureFIFO/FIFOWriteControl ==
  ADC_Data : Inport
  ADC_Valid : Inport  Port=2
  RxStart : Inport  Port=3
  CaptureLength : Inport  Port=4
  DebugMode : Inport  Port=5
  FIFO_Full : Inport  Port=6
  Data Type Conversion : DataTypeConversion
  MATLAB Function : MATLAB Function  TreatAsAtomicUnit=on
  Multiport Switch : MultiPortSwitch  DataPortOrder=Zero-based contiguous  Inputs=2  zeroidx=on
  DataOut : Outport  VectorParamsAs1DForOutWhenUnconnected=off
  DDRCaptureFIFOPush : Outport  Port=2  VectorParamsAs1DForOutWhenUnconnected=off
  DDRCaptureFIFOActive : Outport  Port=3  VectorParamsAs1DForOutWhenUnconnected=off
  FIFODropCount : Outport  Port=4  VectorParamsAs1DForOutWhenUnconnected=off
  wires:
  Data Type Conversion/1 -> Multiport Switch/3
  ADC_Data/1 -> Multiport Switch/2
  DebugMode/1 -> Multiport Switch/1
  Multiport Switch/1 -> DataOut/1
  MATLAB Function/2(DDRCaptureFIFOPush) -> DDRCaptureFIFOPush/1
  FIFO_Full/1 -> MATLAB Function/4(FIFO_Full)
  CaptureLength/1 -> MATLAB Function/3(CaptureLength)
  RxStart/1 -> MATLAB Function/2(RxStart)
  ADC_Valid/1 -> MATLAB Function/1(ADC_Valid)
  MATLAB Function/1(count_out) -> Data Type Conversion/1
  MATLAB Function/3(DDRCaptureFIFOActive) -> DDRCaptureFIFOActive/1
  MATLAB Function/4(FIFODropCount) -> FIFODropCount/1

== system ADC_Capture_4x4_IQ_DDR4/HDL_IP/DDR_Capture_Logic/DataCaptureFIFO/hdl_fwft_fifo ==
  data_i : Inport
  push : Inport  Port=2
  pop : Inport  Port=3
  Compare To Constant : simulink/Logic and Bit Operations/Compare To Constant  relop=>=  const=FIFO_DEPTH-AFULL_THRESH  OutDataTypeStr=boolean
  HDL FIFO : hdlsllib/HDL RAMs/HDL FIFO  fifo_size=FIFO_DEPTH  mode=FWFT  ratio=1  push_msg=Error  pop_msg=Ignore  show_empty=on  show_full=on  show_num=on  LabelModeActiveChoice_Mode=FWFT
      settings: SourceProductName=HDL Coder  SourceProductBaseCode=HD
  Logical Operator1 : Logic  Operator=NOT  IconShape=distinctive  AllPortsSameDT=off  OutDataTypeStr=boolean
  Logical Operator2 : Logic  IconShape=distinctive  AllPortsSameDT=off  OutDataTypeStr=boolean
  data_o : Outport  VectorParamsAs1DForOutWhenUnconnected=off
  empty_o : Outport  Port=2  VectorParamsAs1DForOutWhenUnconnected=off
  num : Outport  Port=3  VectorParamsAs1DForOutWhenUnconnected=off
  full : Outport  Port=4  VectorParamsAs1DForOutWhenUnconnected=off
  afull : Outport  Port=5  VectorParamsAs1DForOutWhenUnconnected=off
  wires:
  Compare To Constant/1 -> afull/1
  HDL FIFO/2 -> empty_o/1
  pop/1 -> HDL FIFO/3
  data_i/1 -> HDL FIFO/1
  push/1 -> Logical Operator2/1
  Logical Operator2/1 -> HDL FIFO/2
  Logical Operator1/1 -> Logical Operator2/2
  HDL FIFO/1 -> data_o/1
  HDL FIFO/3 -> Logical Operator1/1, full/1
  HDL FIFO/4 -> Compare To Constant/1, num/1  "wr_fifo_cnt"

== system ADC_Capture_4x4_IQ_DDR4/HDL_IP/NCO_Transmit1/ScaleIQ and bit concat/For Each IQ Scale ==
  SampleVector : Inport  Partition=on  PartitionDimension=1  PartitionWidth=1  PartitionOffset=0
  Scale_I : Inport  Port=2
  Scale_Q : Inport  Port=3
  Complex to Real-Imag3 : ComplexToRealImag
  Delay16 : Delay  DelayLength=1
  For Each : ForEach  DisableCoverage=on
  Product10 : Product  OutDataTypeStr=Inherit: Same as first input
  Product9 : Product  OutDataTypeStr=Inherit: Same as first input
  ScaledSample_I : Outport  ConcatenationDimension=1  VectorParamsAs1DForOutWhenUnconnected=off
  ScaledSample_Q : Outport  Port=2  ConcatenationDimension=1  VectorParamsAs1DForOutWhenUnconnected=off
  wires:
  Product9/1 -> ScaledSample_I/1
  Complex to Real-Imag3/2 -> Product10/1
  Product10/1 -> ScaledSample_Q/1
  SampleVector/1 -> Delay16/1
  Complex to Real-Imag3/1 -> Product9/1
  Delay16/1 -> Complex to Real-Imag3/1
  Scale_I/1 -> Product9/2
  Scale_Q/1 -> Product10/2

== system ADC_Capture_4x4_IQ_DDR4/HDL_IP/NCO_Transmit1/Vectorized NCO/For Each NCO Vectorized ==
  inc : Inport
  offset : Inport  Port=2  Partition=on  PartitionDimension=1  PartitionWidth=1  PartitionOffset=0
  reset : Inport  Port=3
  Complex to Real-Imag : ComplexToRealImag
  Data Type Conversion : DataTypeConversion  OutDataTypeStr=fixdt(1,16,15)  ConvertRealWorld=Stored Integer (SI)
  For Each : ForEach  DisableCoverage=on
  Gain : Gain  Gain=4  OutDataTypeStr=Inherit: Same as input
  Gain1 : Gain  Gain=4  OutDataTypeStr=Inherit: Same as input
  NCO HDL Optimized1 : dsphdlsigops/NCO HDL Optimized  PhaseIncrementSource=Input port  PhaseIncrement=round(Fo*(2^N)/Fs)  PhaseOffsetSource=Input port  PhaseOffset=0  DitherSource=Property  NumDitherBits=4  PhaseQuantization=off  NumQuantizerAccumulatorBits=12  LUTCompress=on  ResetAction=on  ValidInputPort=off  Waveform=Complex exponential  PhasePort=off  SimulateUsing=Code generation  AccumulatorWL=config.synthesis.N_accumulator  OutputDataType=Binary point scaling  OutputWL=config.synthesis.N_accumulator  OutputFL=-1 + config.synthesis.N_accumulator
      settings: SourceProductName=DSP System Toolbox  SourceProductBaseCode=DS
  Real-Imag to Complex : RealImagToComplex
  Terminator : Terminator
  ComplexChirp Vectorized Samples : Outport  ConcatenationDimension=1
  wires:
  inc/1 -> NCO HDL Optimized1/1  "phase_count_dot"
  NCO HDL Optimized1/1 -> Data Type Conversion/1
  NCO HDL Optimized1/2 -> Terminator/1
  offset/1 -> NCO HDL Optimized1/2
  Data Type Conversion/1 -> Complex to Real-Imag/1
  Complex to Real-Imag/1 -> Gain/1
  Complex to Real-Imag/2 -> Gain1/1
  Gain/1 -> Real-Imag to Complex/1
  Gain1/1 -> Real-Imag to Complex/2
  Real-Imag to Complex/1 -> ComplexChirp Vectorized Samples/1
  reset/1 -> NCO HDL Optimized1/3  "phase_count_dot"

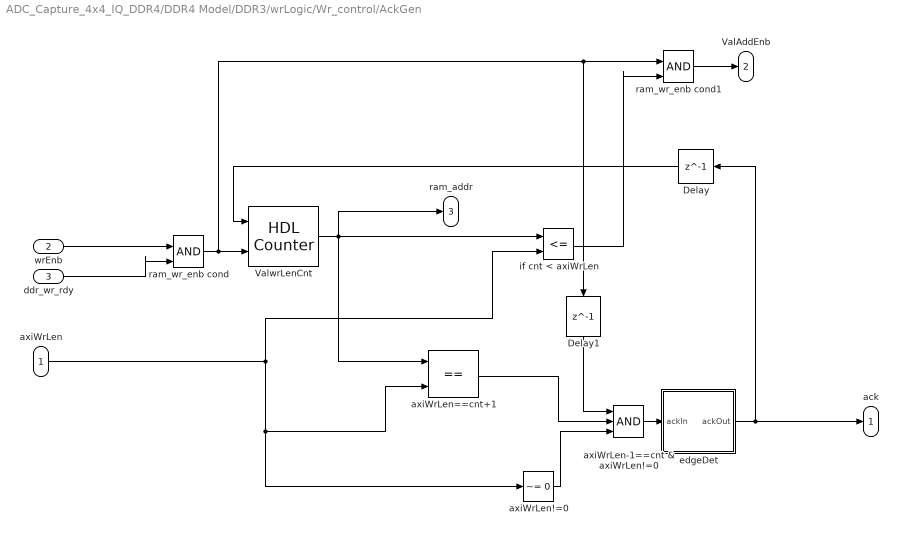
== system ADC_Capture_4x4_IQ_DDR4/DDR4 Model/DDR3/wrLogic/Wr_control/AckGen ==
  axiWrLen : Inport
  wrEnb : Inport  Port=2
  ddr_wr_rdy : Inport  Port=3
  Delay : Delay  DelayLength=1
  Delay1 : Delay  DelayLength=1
  ValwrLenCnt : hdlsllib/Sources/HDL Counter  CountType=Free running  CountInit=0  CountStep=1  CountMax=DDR3_DEPTH  CountFromType=Initial value  CountFrom=0  CountResetPort=on  CountLoadPort=off  CountEnbPort=on  CountDirPort=off  CountDataType=Unsigned  CountWordLen=32  CountFracLen=0  CountSampTime=1
      settings: SourceProductBaseCode=HD
  axiWrLen!=0 : simulink/Logic and Bit Operations/Compare To Constant  relop=~=  const=0  OutDataTypeStr=boolean
  "axiWrLen-1==cnt & axiWrLen!=0 " : Logic  Inputs=3  IconShape=distinctive  AllPortsSameDT=off  OutDataTypeStr=boolean
  axiWrLen==cnt+1 : RelationalOperator  Operator===  OutDataTypeStr=boolean  RndMeth=Nearest
  edgeDet : Subsystem
  if cnt < axiWrLen : RelationalOperator  Operator=<=  OutDataTypeStr=boolean  RndMeth=Nearest
  ram_wr_enb cond : Logic  IconShape=distinctive  AllPortsSameDT=off  OutDataTypeStr=boolean
  ram_wr_enb cond1 : Logic  IconShape=distinctive  AllPortsSameDT=off  OutDataTypeStr=boolean
  ack : Outport  VectorParamsAs1DForOutWhenUnconnected=off
  ValAddEnb : Outport  Port=2  VectorParamsAs1DForOutWhenUnconnected=off
  ram_addr : Outport  Port=3  VectorParamsAs1DForOutWhenUnconnected=off
  wires:
  "axiWrLen-1==cnt & axiWrLen!=0 "/1 -> edgeDet/1(ackIn)
  edgeDet/1(ackOut) -> ack/1, Delay/1
  axiWrLen==cnt+1/1 -> "axiWrLen-1==cnt & axiWrLen!=0 "/2
  axiWrLen!=0/1 -> "axiWrLen-1==cnt & axiWrLen!=0 "/3
  wrEnb/1 -> ram_wr_enb cond/1
  if cnt < axiWrLen/1 -> ram_wr_enb cond1/2
  axiWrLen/1 -> axiWrLen==cnt+1/2, axiWrLen!=0/1, if cnt < axiWrLen/2
  ValwrLenCnt/1 -> axiWrLen==cnt+1/1, if cnt < axiWrLen/1, ram_addr/1
  ddr_wr_rdy/1 -> ram_wr_enb cond/2
  ram_wr_enb cond/1 -> ram_wr_enb cond1/1, Delay1/1, ValwrLenCnt/2
  ram_wr_enb cond1/1 -> ValAddEnb/1
  Delay/1 -> ValwrLenCnt/1
  Delay1/1 -> "axiWrLen-1==cnt & axiWrLen!=0 "/1

== system ADC_Capture_4x4_IQ_DDR4/DDR4 Model/DDR3/wrLogic/Wr_control/AckGen/edgeDet ==
  ackIn : Inport
  " ackIn==1" : simulink/Logic and Bit Operations/Compare To Constant  relop===  const=1  OutDataTypeStr=boolean
  ackIn Posedge Detect : Logic  IconShape=distinctive  AllPortsSameDT=off  OutDataTypeStr=boolean
  ackIn_d1 : Delay  DelayLength=1
  ackIn_d1==0 : simulink/Logic and Bit Operations/Compare To Constant  relop===  const=0  OutDataTypeStr=boolean
  ackOut : Outport  VectorParamsAs1DForOutWhenUnconnected=off
  wires:
  " ackIn==1"/1 -> ackIn Posedge Detect/2
  ackIn_d1==0/1 -> ackIn Posedge Detect/1
  ackIn Posedge Detect/1 -> ackOut/1
  ackIn_d1/1 -> ackIn_d1==0/1
  ackIn/1 -> " ackIn==1"/1, ackIn_d1/1

== matlab function ADC_Capture_4x4_IQ_DDR4/HDL_IP/System Controller ==
  data: cpi_start input; tx_active output; cpi_len input; pulse_width input; pri input; rx_active output; rng_gate_delay input; rx_start output; prf_rst output; rng_swath_length input
function [tx_active, rx_active, rx_start, prf_rst] = ...
    sys_ctrl(cpi_start, cpi_len, pulse_width, pri, rng_gate_delay, rng_swath_length)

[tx_active, rx_active, rx_start, prf_rst] = ...
    controller.system_controller(cpi_start, cpi_len, pulse_width, pri, rng_gate_delay, rng_swath_length)

end

== matlab function ADC_Capture_4x4_IQ_DDR4/DDR4 Model/DDR3/load_init_data ==
  data: load_done output; ram_wr_data output; axi_wr_data input; axi_wr_add input; axi_wr_val input; ram_wr_add output; ram_wr_enb output boolean; INIT_ADDR parameter; DDR3_DEPTH parameter; INIT_DDR3 parameter; INIT_DATA parameter
function [load_done,ram_wr_data,ram_wr_add,ram_wr_enb] = load_init(axi_wr_data,axi_wr_add,axi_wr_val, INIT_ADDR, DDR3_DEPTH, INIT_DDR3,INIT_DATA)

%%%%%%%%%%%%%%%%%%%%%%%%%%%%%%%%%%%%%%%%%%%%%%%%%%%%%%
% Create persistent variables (registers)
persistent reg_ram_wr_add;
if(isempty(reg_ram_wr_add))
    reg_ram_wr_add = fi(0,0,32,0);
end

ram_wr_data = cast(0,'like',axi_wr_data);

persistent reg_ram_wr_data;
if(isempty(reg_ram_wr_data))
    reg_ram_wr_data =cast(0,'like',axi_wr_data);% fi(0,1,ddrWidth,0);
end

persistent reg_ram_wr_data_d1;
if(isempty(reg_ram_wr_data_d1))
    reg_ram_wr_data_d1 = cast(0,'like',axi_wr_data);%
end


persistent state;
if(isempty(state))
    state = fi(0, 0, 3, 0);
end


persistent reg_ram_wr_enb;
if(isempty(reg_ram_wr_enb))
    reg_ram_wr_enb = false;
end

persistent reg_ram_wr_enb_d1;
if(isempty(reg_ram_wr_enb_d1))
    reg_ram_wr_enb_d1 = false;
end

persistent reg_init_data;
if(isempty(reg_init_data))
    reg_init_data = cast(zeros(1,DDR3_DEPTH),'like',axi_wr_data);% fi(zeros(1,DDR3_DEPTH),1,ddrWidth,0);
end

%%%%%%%%%%%%%%%%%%%%%%%%%%%%%%%%%%%%%%%%%%%%%%%%%%
% State Memory Encoding
INIT_ST    = fi(0, 0, 3, 0);
LOAD_START = fi(1, 0, 3, 0);
LOAD_PROG  = fi(3, 0, 3, 0);
LOAD_DONE  = fi(2, 0, 3, 0);
DATA_ST    = fi(6, 0, 3, 0);


% init phase states
% 1. Every state MUST assign every output value
% 2. Use explicit data type always
switch (state)
    case INIT_ST
       
        reg_ram_wr_add = fi(0,0,32,0);%uint32(0);
        reg_ram_wr_data =  cast(0,'like',axi_wr_data);%fi(0,1,ddrWidth,0);%int32(0);
        reg_ram_wr_enb = false;
        load_done = false;
        
    case LOAD_START
        
        reg_ram_wr_add = fi(INIT_ADDR,0,32,0);
        reg_ram_wr_data =  cast(reg_init_data(1,reg_ram_wr_add+1),'like',axi_wr_data);%fi(reg_init_data(1,reg_ram_wr_add+1),1,ddrWidth,0);%int32(INIT_DATA);
        reg_ram_wr_enb = true;
        load_done = false;
    case LOAD_PROG
        
        
        reg_ram_wr_add = fi(reg_ram_wr_add+1,0,32,0);
        reg_ram_wr_data =  cast(reg_init_data(1,reg_ram_wr_add+1),'like',axi_wr_data);%fi(reg_init_data(1,reg_ram_wr_add+1),1,ddrWidth,0);%int32(INIT_DATA);
        reg_ram_wr_enb = true;
        load_done = false;
    case LOAD_DONE
      
        reg_ram_wr_add = fi(reg_ram_wr_add,0,32,0);
       % reg_ram_wr_data = reg_ram_wr_data;%fi(reg_ram_wr_data,1,ddrWidth,0);
        reg_ram_wr_enb = true;
        load_done = true;
    case DATA_ST    
        %external (AXI ) inputs
        reg_ram_wr_add = fi(axi_wr_add,0,32,0);
        reg_ram_wr_data =  axi_wr_data;%fi(axi_wr_data,1,ddrWidth,0);
        reg_ram_wr_enb = axi_wr_val;
        load_done = true;
    otherwise
        
        reg_ram_wr_add = fi(0,0,32,0);
        reg_ram_wr_data =  cast(0,'like',axi_wr_data);%fi(0,1,ddrWidth,0);
        reg_ram_wr_enb = false;
        load_done = false;
end

ram_wr_add = fi(reg_ram_wr_add,0,32,0);
%ram_wr_data = reg_ram_wr_data;

if(load_done == true)
   ram_wr_data = cast(reg_ram_wr_data_d1,'like',axi_wr_data);%fi(reg_ram_wr_data_d1,1,ddrWidth,0);%reg_ram_wr_data_d1;
else
   ram_wr_data = cast(reg_ram_wr_data_d1,'like',axi_wr_data);%fi(reg_ram_wr_data_d1,1,ddrWidth,0);%reg_ram_wr_data;   
end


if(load_done == true)
   ram_wr_enb = reg_ram_wr_enb_d1;
else
   ram_wr_enb = reg_ram_wr_enb;   
end


if(load_done == false)
   reg_init_data = cast(INIT_DATA,'like',axi_wr_data);%fi(INIT_DATA,1,ddrWidth,0);%reg_ram_wr_data;   
end

reg_ram_wr_enb_d1 = reg_ram_wr_enb;
reg_ram_wr_data_d1 = reg_ram_wr_data;%fi(reg_ram_wr_data,1,ddrWidth,0);%int32(reg_ram_wr_data);
% Next State Logic
switch (state)
    case INIT_ST
        
        if ( INIT_DDR3 == true)
            nextState = LOAD_START;
        else
            nextState = DATA_ST;
        end
    case LOAD_START
            nextState = LOAD_PROG;
    case LOAD_PROG
        if(fi(ram_wr_add,0,32,0)==fi(DDR3_DEPTH-1,0,32,0))
            nextState = LOAD_DONE;
        else
            nextState = LOAD_PROG;
        end
    case LOAD_DONE
            nextState = DATA_ST;
    case DATA_ST
            nextState = DATA_ST; 
    otherwise
        nextState = INIT_ST;
end

state = nextState;

end
